simulink model "pibit_completo_sem_obs_2025"  (R2025a)
settings: Solver=VariableStepAuto  StartTime=0.0  StopTime=40  RelTol=1e-3
values from neighbouring files (symbols this model uses):
  bp = 5    [parametros_suspensao_completo_pibit.m]    (also in parametros_suspensao_completo_pibit_final.m)
  bs = 10    [parametros_suspensao_completo_pibit.m]    (also in parametros_suspensao_completo_pibit_final.m)
  g = 9.81    [parametros_suspensao_completo_pibit.m]    (also in parametros_suspensao_completo_pibit_final.m)
  I = 5.6e-4    (= 0.00056)    [parametros_suspensao_completo_pibit.m]    (also in parametros_suspensao_completo_pibit_final.m)
  I_carroceria = (1/12) * m_carroceria * (L^2 + H^2)    (= 0.0082936384875)    [parametros_suspensao_completo_pibit_final.m]
  kp = 1000    [parametros_suspensao_completo_pibit.m]    (also in parametros_suspensao_completo_pibit_final.m)
  ks = 200    [parametros_suspensao_completo_pibit.m]    (also in parametros_suspensao_completo_pibit_final.m)
  M = [ ... (first row only)    [aprimorado_matlab_function_matriz_transformacao.m]    (also in bloco_matriz_tranformacao_pibit_final.m; bloco_matriz_tranformacao_pibit_semifinal.m; bloco_transposta_matriz_transformacao.m; matlab_function_matriz_transformacao.m)
  m_carroceria = 0.598725    [parametros_suspensao_completo_pibit_final.m]
  M_transposta = M'    [bloco_transposta_matriz_transformacao.m]    (also in parametros_suspensao_completo_pibit_final.m = [1  0  1  0  1)
  massa_nao_suspensa = 200/1000    (= 0.2)    [parametros_suspensao_completo_pibit.m]    (also in parametros_suspensao_completo_pibit_final.m)
  Vv = 5    [parametros_suspensao_completo_pibit_final.m]
  z0_carroceria = 0.12    [parametros_suspensao_completo_pibit_final.m]
  z0_roda = 0.04    [parametros_suspensao_completo_pibit_final.m]

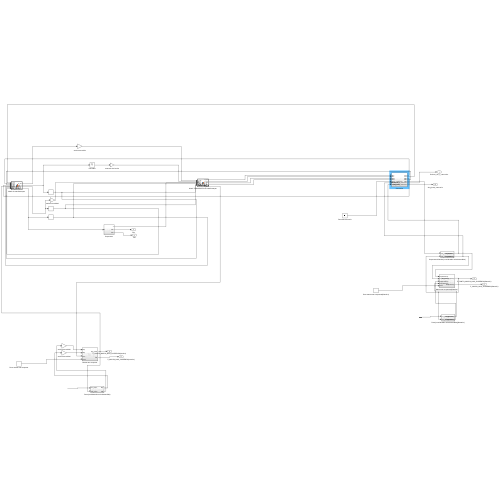
[thumbnail: Simulink's stored preview of the top-level diagram]
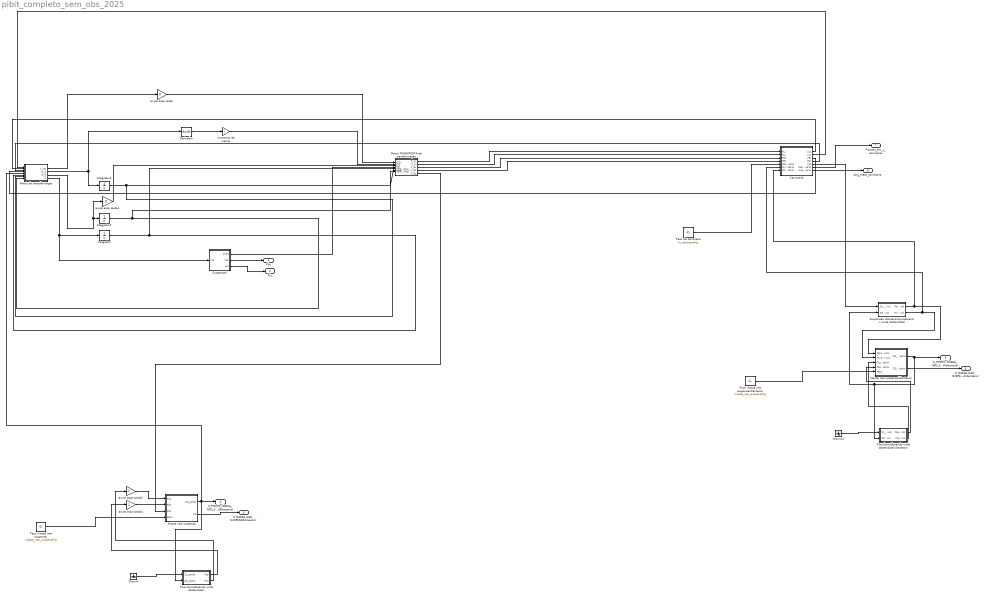
== system pibit_completo_sem_obs_2025 ==
  Carroceria : Subsystem
  Derivador : Derivative
  Ground : Ground
  Ground1 : Ground
  Integrator : Integrator
  Integrator2 : Integrator
  Integrator3 : Integrator
  Massa nao suspensa : Subsystem
  Massa nao suspensa(dianteira) : Subsystem
  Matris TRANSPOSTA de transformaçao : MATLAB Function  TreatAsAtomicUnit=on
  Matriz de transformaçao : MATLAB Function  TreatAsAtomicUnit=on
  Peso da carroceria : Constant  Value=m_carroceria*g
  Peso massa nao suspensa : Constant  Value=massa_nao_suspensa*g
  Peso massa nao suspensa(dianteira) : Constant  Value=massa_nao_suspensa*g
  Pneu(considerando mola destendida) : Subsystem
  Pneu(considerando mola destendida)(dianteiro) : Subsystem
  Suspensao : Subsystem
  Suspensao dianteira(considerando mola destendida) : Subsystem
  anula essa saida : Gain  Gain=0
  anula essa saida1 : Gain  Gain=0
  anula essa saida3 : Gain
  anula essa saida4 : Gain
  momento de inercia : Gain  Gain=I
  Fbs : Outport
  Fks : Outport  Port=2
  Z_MASSA_NAO_SUSPENSA(traseiro) : Outport  Port=3
  Z_PONTO_MASSA_NAO_SUSPENSA(traseiro) : Outport  Port=4
  Z_MASSA_NAO_SUSPENSA(dianteiro) : Outport  Port=5
  Z_PONTO_MASSA_NAO_SUSPENSA(dianteiro) : Outport  Port=6
  Posicao_em_z_carroceria : Outport  Port=7
  Ang_theta_carroceria : Outport  Port=8
  wires:
  Derivador/1 -> momento de inercia/1
  anula essa saida1/1 -> Matris TRANSPOSTA de transformaçao/3(M_s)
  Suspensao/1(Out1) -> Matris TRANSPOSTA de transformaçao/4(F_s)
  Matris TRANSPOSTA de transformaçao/1(F_Lx) -> Carroceria/1(FLx)
  Suspensao dianteira(considerando mola destendida)/2(Fk(dianteiro)) -> Carroceria/6(Fk(dianteiro)), Massa nao suspensa(dianteira)/2(Fk(dianteiro)2)
  Integrator/1 -> Matris TRANSPOSTA de transformaçao/5(delta_BETA_1), Matriz de transformaçao/6(delta_BETA_1)
  Pneu(considerando mola destendida)(dianteiro)/2(Fkp(dianteiro)) -> Massa nao suspensa(dianteira)/3(Fkp(dianteiro))
  Carroceria/3(VEz) -> Matriz de transformaçao/4(V_Ez)
  anula essa saida4/1 -> Massa nao suspensa/2(Fbp)
  Peso massa nao suspensa/1 -> Massa nao suspensa/4(Peso)
  Carroceria/2(VLx) -> Matriz de transformaçao/1(V_Lx)
  Massa nao suspensa(dianteira)/1(ZG_ponto(dianteiro)) -> Z_PONTO_MASSA_NAO_SUSPENSA(dianteiro)/1, Pneu(considerando mola destendida)(dianteiro)/2(ZG_ponto(dianteiro)), Suspensao dianteira(considerando mola destendida)/2(ZG_ponto(dianteiro))
  Matriz de transformaçao/1(V_Gx) -> anula essa saida/1
  Matris TRANSPOSTA de transformaçao/5(F_Gz) -> Massa nao suspensa/3(FGz)
  anula essa saida/1 -> Matris TRANSPOSTA de transformaçao/1(F_Gx)
  Carroceria/7(Ang_theta_carroceria) -> Ang_theta_carroceria/1
  momento de inercia/1 -> Matris TRANSPOSTA de transformaçao/2(M_b)
  Carroceria/5(VAz) -> Suspensao dianteira(considerando mola destendida)/1(ZA_ponto(dianteiro))
  Massa nao suspensa/2(ZG) -> Z_MASSA_NAO_SUSPENSA(traseiro)/1
  Matris TRANSPOSTA de transformaçao/3(F_Ex) -> Carroceria/3(FEx)
  Matris TRANSPOSTA de transformaçao/2(F_Lz) -> Carroceria/2(FLz)
  Carroceria/6(Posicao_em_z_carroceria) -> Posicao_em_z_carroceria/1
  Suspensao/3(Fks) -> Fks/1
  Carroceria/4(VEx) -> Matriz de transformaçao/3(V_Ex)
  anula essa saida3/1 -> Massa nao suspensa/1(Fkp)
  Matris TRANSPOSTA de transformaçao/4(F_Ez) -> Carroceria/4(FEz)
  Pneu(considerando mola destendida)/2(Fkp) -> anula essa saida3/1
  Carroceria/1(VLz) -> Matriz de transformaçao/2(V_Lz)
  Peso massa nao suspensa(dianteira)/1 -> Massa nao suspensa(dianteira)/5(Peso)
  Peso da carroceria/1 -> Carroceria/5(Peso_carroceria)
  Matriz de transformaçao/4(BETA_1_PONTO) -> Suspensao/1(In1), Integrator/1
  Integrator3/1 -> Matriz de transformaçao/7(delta_BETA_2), Matris TRANSPOSTA de transformaçao/6(delta_BETA_2)
  Matriz de transformaçao/2(W_b) -> Derivador/1, Integrator3/1
  Pneu(considerando mola destendida)/1(Fbp) -> anula essa saida4/1
  Massa nao suspensa/1(ZG_ponto) -> Z_PONTO_MASSA_NAO_SUSPENSA(traseiro)/1, Pneu(considerando mola destendida)/2(ZG_ponto), Matriz de transformaçao/5(V_Gz)
  Massa nao suspensa(dianteira)/2(ZG(dianteiro)) -> Z_MASSA_NAO_SUSPENSA(dianteiro)/1
  Suspensao/2(Fbs) -> Fbs/1
  Pneu(considerando mola destendida)(dianteiro)/1(Fbp(dianteiro)) -> Massa nao suspensa(dianteira)/4(Fbp(dianteiro))
  Integrator2/1 -> Matriz de transformaçao/8(delta_BETA_3), Matris TRANSPOSTA de transformaçao/7(delta_BETA_3)
  Suspensao dianteira(considerando mola destendida)/1(Fb(dianteiro)) -> Carroceria/7(Fb(dianteiro)), Massa nao suspensa(dianteira)/1(Fb(dianteiro)1)
  Matriz de transformaçao/3(W_s) -> anula essa saida1/1, Integrator2/1
  Ground/1 -> Pneu(considerando mola destendida)/1(Z1_ponto)
  Ground1/1 -> Pneu(considerando mola destendida)(dianteiro)/1(Z1_ponto(dianteiro))

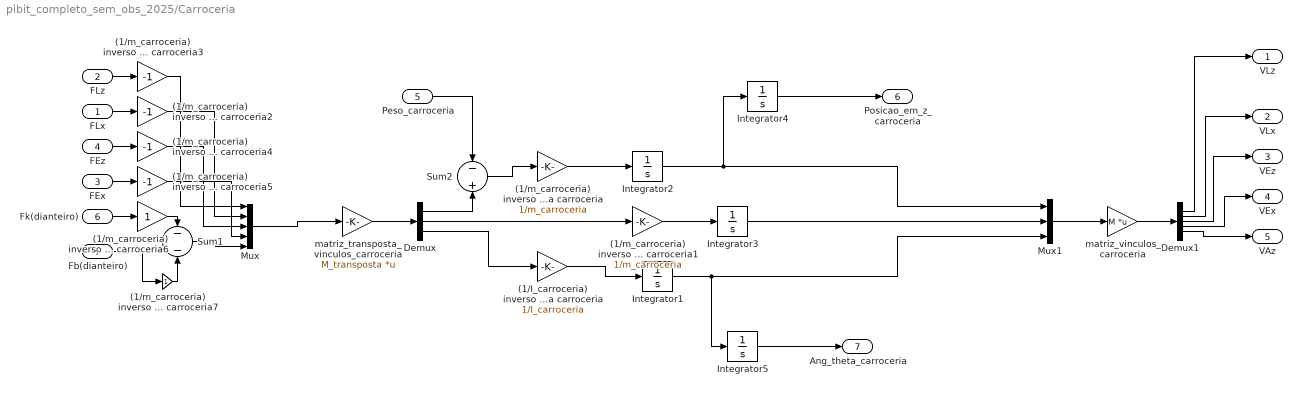
== system pibit_completo_sem_obs_2025/Carroceria ==
  FLx : Inport
  FLz : Inport  Port=2
  FEx : Inport  Port=3
  FEz : Inport  Port=4
  Peso_carroceria : Inport  Port=5
  Fk(dianteiro) : Inport  Port=6
  Fb(dianteiro) : Inport  Port=7
  (1/I_carroceria) inverso do momento de inercia da carroceria : Gain  Gain=1/I_carroceria
  (1/m_carroceria) inverso da massa da carroceria : Gain  Gain=1/m_carroceria
  (1/m_carroceria) inverso da massa da carroceria1 : Gain  Gain=1/m_carroceria
  (1/m_carroceria) inverso da massa da carroceria{2..5} (4 alike) : Gain  Gain=-1
  (1/m_carroceria) inverso da massa da carroceria6 : Gain
  (1/m_carroceria) inverso da massa da carroceria7 : Gain
  Demux : Demux  Outputs=3
  Demux1 : Demux  Outputs=5
  Integrator1 : Integrator
  Integrator2 : Integrator
  Integrator3 : Integrator  InitialCondition=Vv
  Integrator4 : Integrator  InitialCondition=z0_carroceria
  Integrator5 : Integrator
  Mux : Mux  Inputs=5
  Mux1 : Mux  Inputs=3
  Sum1 : Sum  Inputs=--
  Sum2 : Sum  Inputs=-+
  matriz_transposta_vinculos_carroceria : Gain  Gain=M_transposta  Multiplication=Matrix(K*u) (u vector)
  matriz_vinculos_carroceria : Gain  Gain=M  Multiplication=Matrix(K*u) (u vector)
  VLz : Outport
  VLx : Outport  Port=2
  VEz : Outport  Port=3
  VEx : Outport  Port=4
  VAz : Outport  Port=5
  Posicao_em_z_carroceria : Outport  Port=6
  Ang_theta_carroceria : Outport  Port=7
  wires:
  Fk(dianteiro)/1 -> (1/m_carroceria) inverso da massa da carroceria6/1
  Fb(dianteiro)/1 -> (1/m_carroceria) inverso da massa da carroceria7/1
  FLz/1 -> (1/m_carroceria) inverso da massa da carroceria3/1
  FLx/1 -> (1/m_carroceria) inverso da massa da carroceria2/1
  FEz/1 -> (1/m_carroceria) inverso da massa da carroceria4/1
  FEx/1 -> (1/m_carroceria) inverso da massa da carroceria5/1
  Sum1/1 -> Mux/5
  Mux/1 -> matriz_transposta_vinculos_carroceria/1
  matriz_transposta_vinculos_carroceria/1 -> Demux/1
  Peso_carroceria/1 -> Sum2/1
  Demux/1 -> Sum2/2
  Sum2/1 -> (1/m_carroceria) inverso da massa da carroceria/1
  (1/m_carroceria) inverso da massa da carroceria/1 -> Integrator2/1
  Demux/2 -> (1/m_carroceria) inverso da massa da carroceria1/1
  Demux/3 -> (1/I_carroceria) inverso do momento de inercia da carroceria/1
  (1/I_carroceria) inverso do momento de inercia da carroceria/1 -> Integrator1/1
  (1/m_carroceria) inverso da massa da carroceria1/1 -> Integrator3/1
  Integrator2/1 -> Integrator4/1, Mux1/1
  Mux1/1 -> matriz_vinculos_carroceria/1
  matriz_vinculos_carroceria/1 -> Demux1/1
  Demux1/1 -> VLz/1
  Demux1/2 -> VLx/1
  Demux1/3 -> VEz/1
  Demux1/4 -> VEx/1
  Demux1/5 -> VAz/1
  Integrator1/1 -> Integrator5/1, Mux1/3
  (1/m_carroceria) inverso da massa da carroceria3/1 -> Mux/1
  (1/m_carroceria) inverso da massa da carroceria2/1 -> Mux/2
  (1/m_carroceria) inverso da massa da carroceria4/1 -> Mux/3
  (1/m_carroceria) inverso da massa da carroceria5/1 -> Mux/4
  (1/m_carroceria) inverso da massa da carroceria6/1 -> Sum1/1
  (1/m_carroceria) inverso da massa da carroceria7/1 -> Sum1/2
  Integrator3/1 -> Mux1/2
  Integrator4/1 -> Posicao_em_z_carroceria/1
  Integrator5/1 -> Ang_theta_carroceria/1

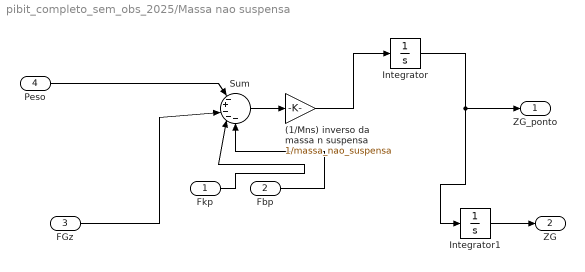
== system pibit_completo_sem_obs_2025/Massa nao suspensa ==
  Fkp : Inport
  Fbp : Inport  Port=2
  FGz : Inport  Port=3
  Peso : Inport  Port=4
  (1/Mns) inverso da massa n suspensa : Gain  Gain=1/massa_nao_suspensa
  Integrator : Integrator
  Integrator1 : Integrator  InitialCondition=z0_roda
  Sum : Sum  Inputs=|-+---
  ZG_ponto : Outport
  ZG : Outport  Port=2
  wires:
  Integrator/1 -> Integrator1/1, ZG_ponto/1
  Fbp/1 -> Sum/5
  Fkp/1 -> Sum/4
  (1/Mns) inverso da massa n suspensa/1 -> Integrator/1
  Sum/1 -> (1/Mns) inverso da massa n suspensa/1
  FGz/1 -> Sum/3
  Peso/1 -> Sum/1
  Integrator1/1 -> ZG/1

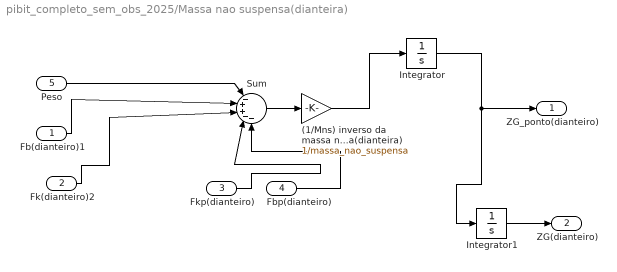
== system pibit_completo_sem_obs_2025/Massa nao suspensa(dianteira) ==
  Fb(dianteiro)1 : Inport
  Fk(dianteiro)2 : Inport  Port=2
  Fkp(dianteiro) : Inport  Port=3
  Fbp(dianteiro) : Inport  Port=4
  Peso : Inport  Port=5
  (1/Mns) inverso da massa nao suspensa(dianteira) : Gain  Gain=1/massa_nao_suspensa
  Integrator : Integrator
  Integrator1 : Integrator  InitialCondition=z0_roda
  Sum : Sum  Inputs=|-++--
  ZG_ponto(dianteiro) : Outport
  ZG(dianteiro) : Outport  Port=2
  wires:
  Integrator/1 -> Integrator1/1, ZG_ponto(dianteiro)/1
  Fbp(dianteiro)/1 -> Sum/5
  Fkp(dianteiro)/1 -> Sum/4
  (1/Mns) inverso da massa nao suspensa(dianteira)/1 -> Integrator/1
  Sum/1 -> (1/Mns) inverso da massa nao suspensa(dianteira)/1
  Peso/1 -> Sum/1
  Integrator1/1 -> ZG(dianteiro)/1
  Fb(dianteiro)1/1 -> Sum/2
  Fk(dianteiro)2/1 -> Sum/3

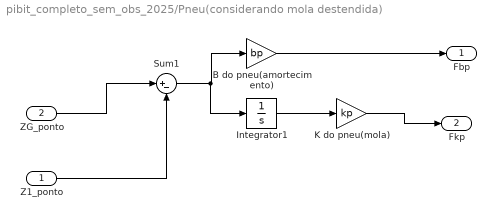
== system pibit_completo_sem_obs_2025/Pneu(considerando mola destendida) ==
  Z1_ponto : Inport
  ZG_ponto : Inport  Port=2
  B do pneu(amortecimento) : Gain  Gain=bp
  Integrator1 : Integrator
  K do pneu(mola) : Gain  Gain=kp
  Sum1 : Sum  Inputs=|+-
  Fbp : Outport
  Fkp : Outport  Port=2
  wires:
  Z1_ponto/1 -> Sum1/2
  ZG_ponto/1 -> Sum1/1
  Sum1/1 -> Integrator1/1, B do pneu(amortecimento)/1
  K do pneu(mola)/1 -> Fkp/1
  B do pneu(amortecimento)/1 -> Fbp/1
  Integrator1/1 -> K do pneu(mola)/1

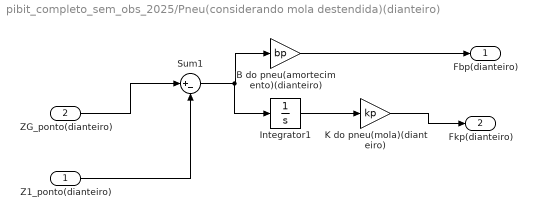
== system pibit_completo_sem_obs_2025/Pneu(considerando mola destendida)(dianteiro) ==
  Z1_ponto(dianteiro) : Inport
  ZG_ponto(dianteiro) : Inport  Port=2
  B do pneu(amortecimento)(dianteiro) : Gain  Gain=bp
  Integrator1 : Integrator
  K do pneu(mola)(dianteiro) : Gain  Gain=kp
  Sum1 : Sum  Inputs=|+-
  Fbp(dianteiro) : Outport
  Fkp(dianteiro) : Outport  Port=2
  wires:
  Z1_ponto(dianteiro)/1 -> Sum1/2
  ZG_ponto(dianteiro)/1 -> Sum1/1
  Sum1/1 -> Integrator1/1, B do pneu(amortecimento)(dianteiro)/1
  K do pneu(mola)(dianteiro)/1 -> Fkp(dianteiro)/1
  B do pneu(amortecimento)(dianteiro)/1 -> Fbp(dianteiro)/1
  Integrator1/1 -> K do pneu(mola)(dianteiro)/1

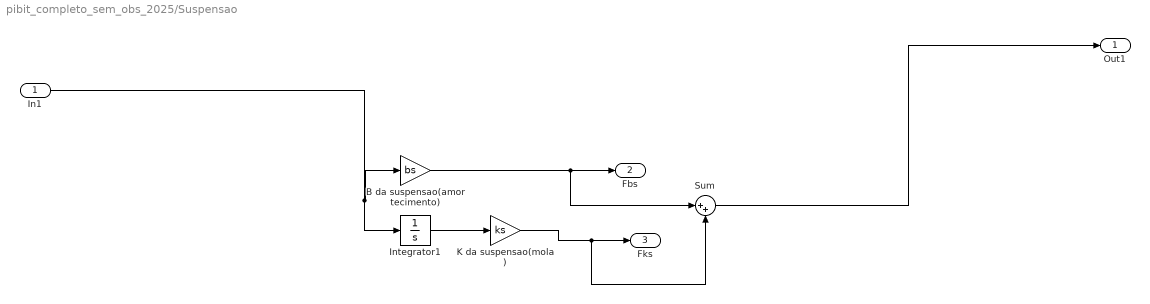
== system pibit_completo_sem_obs_2025/Suspensao ==
  In1 : Inport
  B da suspensao(amortecimento) : Gain  Gain=bs
  Integrator1 : Integrator
  K da suspensao(mola) : Gain  Gain=ks
  Sum : Sum  Inputs=|++
  Out1 : Outport
  Fbs : Outport  Port=2
  Fks : Outport  Port=3
  wires:
  K da suspensao(mola)/1 -> Fks/1, Sum/2
  Sum/1 -> Out1/1
  B da suspensao(amortecimento)/1 -> Fbs/1, Sum/1
  Integrator1/1 -> K da suspensao(mola)/1
  In1/1 -> Integrator1/1, B da suspensao(amortecimento)/1

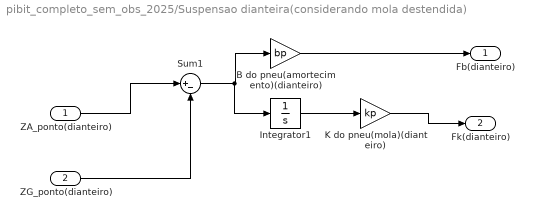
== system pibit_completo_sem_obs_2025/Suspensao dianteira(considerando mola destendida) ==
  ZA_ponto(dianteiro) : Inport
  ZG_ponto(dianteiro) : Inport  Port=2
  B do pneu(amortecimento)(dianteiro) : Gain  Gain=bp
  Integrator1 : Integrator
  K do pneu(mola)(dianteiro) : Gain  Gain=kp
  Sum1 : Sum  Inputs=|+-
  Fb(dianteiro) : Outport
  Fk(dianteiro) : Outport  Port=2
  wires:
  ZG_ponto(dianteiro)/1 -> Sum1/2
  ZA_ponto(dianteiro)/1 -> Sum1/1
  Sum1/1 -> Integrator1/1, B do pneu(amortecimento)(dianteiro)/1
  K do pneu(mola)(dianteiro)/1 -> Fk(dianteiro)/1
  B do pneu(amortecimento)(dianteiro)/1 -> Fb(dianteiro)/1
  Integrator1/1 -> K do pneu(mola)(dianteiro)/1

== matlab function pibit_completo_sem_obs_2025/Matris TRANSPOSTA de transformaçao ==
  data: F_Gx input; F_Lx output; M_b input; M_s input; F_s input; F_Lz output; F_Ex output; F_Ez output; F_Gz output; delta_BETA_1 input; delta_BETA_2 input; delta_BETA_3 input

function [F_Lx, F_Lz, F_Ex, F_Ez, F_Gz] = minhaFuncaoForcas( ...
    F_Gx, M_b, M_s, F_s, delta_BETA_1, delta_BETA_2, delta_BETA_3)

    % Valores nominais iniciais
    BETA_1_0 = 0.055;
    BETA_2_0 = 2.6;
    BETA_3_0 = 2.2;

    % Limites físicos dos parâmetros
    BETA_1_min = 0.05465;
    BETA_1_max = 0.0589;
    BETA_2_min = 2.591;
    BETA_2_max = 2.729;
    BETA_3_min = 2.168;
    BETA_3_max = 2.264;

    % Atualização com limite (clamping)
    BETA_1 = min(max(BETA_1_0 + delta_BETA_1, BETA_1_min), BETA_1_max);
    BETA_2 = min(max(BETA_2_0 + delta_BETA_2, BETA_2_min), BETA_2_max);
    BETA_3 = min(max(BETA_3_0 + delta_BETA_3, BETA_3_min), BETA_3_max);

    % Constantes fixas
    GAMA = 0.380;
    R_1 = 0.091782;
    R_2 = 0.048414;

    % Matriz M atualizada
    M = [
        0, 0, 1, -tan(BETA_2), tan(BETA_2);
        0, 0, 0, 1 / (R_1 * cos(BETA_2)), -1 / (R_1 * cos(BETA_2));
        sin(BETA_3) / BETA_1, cos(BETA_3) / BETA_1, -sin(BETA_3) / BETA_1, ...
        (R_2 * cos(BETA_2 + GAMA - BETA_3) / (R_1 * cos(BETA_2) * BETA_1)) - cos(BETA_3) / BETA_1, ...
        -R_2 * cos(BETA_2 + GAMA - BETA_3) / (R_1 * cos(BETA_2) * BETA_1);
        -cos(BETA_3), sin(BETA_3), cos(BETA_3), ...
        (R_2 * sin(-(BETA_2 + GAMA) + BETA_3) / (R_1 * cos(BETA_2))) - sin(BETA_3), ...
        R_2 * sin((BETA_2 + GAMA) - BETA_3) / (R_1 * cos(BETA_2))
    ];

    % Matriz transposta
    M_transposta = M';

    % Cálculo do resultado
    resultado = M_transposta * [F_Gx; M_b; M_s; F_s];

    % Saídas
    F_Lx = resultado(1);
    F_Lz = resultado(2);
    F_Ex = resultado(3);
    F_Ez = resultado(4);
    F_Gz = resultado(5);
end

== matlab function pibit_completo_sem_obs_2025/Matriz de transformaçao ==
  data: V_Lx input; V_Gx output; V_Lz input; V_Ex input; V_Ez input; V_Gz input; W_b output; W_s output; BETA_1_PONTO output; delta_BETA_1 input; delta_BETA_2 input; delta_BETA_3 input
function [V_Gx, W_b, W_s, BETA_1_PONTO] = fcn( ...
    V_Lx, V_Lz, V_Ex, V_Ez, V_Gz, ...
    delta_BETA_1, delta_BETA_2, delta_BETA_3)

% Valores nominais (iniciais)
BETA_1_0 = 0.055;
BETA_2_0 = 2.6;
BETA_3_0 = 2.2;

% Limites físicos dos parâmetros
BETA_1_min = 0.05465;
BETA_1_max = 0.0589;
BETA_2_min = 2.591;
BETA_2_max = 2.729;
BETA_3_min = 2.168;
BETA_3_max = 2.264;

% Atualização dos parâmetros
BETA_1 = min(max(BETA_1_0 + delta_BETA_1, BETA_1_min), BETA_1_max);
BETA_2 = min(max(BETA_2_0 + delta_BETA_2, BETA_2_min), BETA_2_max);
BETA_3 = min(max(BETA_3_0 + delta_BETA_3, BETA_3_min), BETA_3_max);

% Constantes
GAMA = 0.380;
R_1 = 0.091782;
R_2 = 0.048414;

% Matriz M
M = [
    0, 0, 1, -tan(BETA_2), tan(BETA_2);
    0, 0, 0, 1 / (R_1 * cos(BETA_2)), -1 / (R_1 * cos(BETA_2));
    sin(BETA_3) / BETA_1, cos(BETA_3) / BETA_1, -sin(BETA_3) / BETA_1, ...
    (R_2 * cos(BETA_2 + GAMA - BETA_3) / (R_1 * cos(BETA_2) * BETA_1)) - cos(BETA_3) / BETA_1, ...
    -R_2 * cos(BETA_2 + GAMA - BETA_3) / (R_1 * cos(BETA_2) * BETA_1);
    -cos(BETA_3), sin(BETA_3), cos(BETA_3), ...
    (R_2 * sin(-(BETA_2 + GAMA) + BETA_3) / (R_1 * cos(BETA_2))) - sin(BETA_3), ...
    R_2 * sin((BETA_2 + GAMA) - BETA_3) / (R_1 * cos(BETA_2))
];

entrada = [V_Lx; V_Lz; V_Ex; V_Ez; V_Gz];
resultado = M * entrada;

% Saídas
V_Gx         = resultado(1);
W_b          = resultado(2);
W_s          = resultado(3);
BETA_1_PONTO = resultado(4);
